simulink model "analysis1"  (Simulink 9.0)
settings: Solver=VariableStepAuto  StartTime=0.0  StopTime=0.1  RelTol=1e-3
libraries: dspstat3 x5
settings Model: Creator=CQC  LastModifiedBy=CQC
settings DataIOCC: SaveFormat=Dataset
settings OptimizationCC: LifeSpan=auto
settings DebuggingCC: UnderspecifiedInitializationDetection=Simplified  MergeDetectMultiDrivingBlocksExec=error  SFUnexpectedBacktrackingDiag=error  SFNoUnconditionalDefaultTransitionDiag=error  SFExecutionAtInitializationDiag=warning
settings HardwareCC: ProdBitPerPointer=64  ProdBitPerSizeT=64  ProdBitPerPtrDiffT=64  ProdLargestAtomicFloat=Float  ProdIntDivRoundTo=Zero  ProdEndianess=LittleEndian  ProdWordSize=64  ProdHWDeviceType=Intel->x86-64 (Windows64)
settings ModelReferenceCC: PropagateSignalLabelsOutOfModel=on
settings CodeAppCC: StateflowObjectComments=off
settings GRTTargetCC: TargetLangStandard=C99 (ISO)
settings ConfigComp: CovMetricSettings=dwe  CovHtmlReporting=off  CovSaveCumulativeToWorkspaceVar=off  CovSaveSingleToWorkspaceVar=off  CovExternalEMLEnable=on

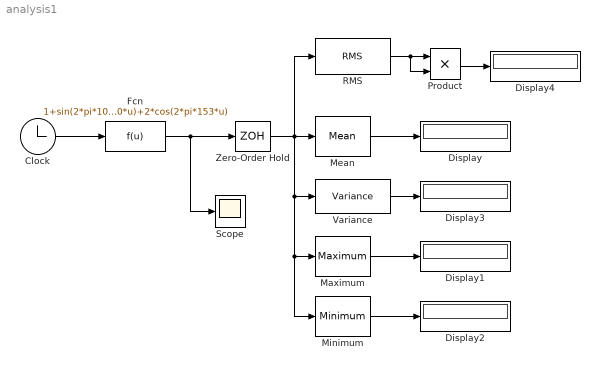
== system analysis1 ==
  Clock : Clock
      settings: Decimation=10000
  Display{,1..4} (5 alike) : Display
  Fcn : Fcn  Expr=1+sin(2*pi*100*u)+2*cos(2*pi*153*u)
  Maximum : dspstat3/Maximum  operation=maximum  fcn=Running  indexBase=One  operateOver=Each column  Dimension=1  InputProcessing=Columns as channels (frame based)  reset=None  roiEnable=off  roiType=Rectangles  roiPortion=Entire ROI  roiOutput=Individual statistics for each ROI  roiFlag=off  roundingMode=Floor  overflowMode=off  accumDataTypeStr=Inherit: Same as product output  accumLastDataTypeStr=Inherit: Same as product output
  Mean : dspstat3/Mean  run=on  reset_popup=None  InputProcessing=Columns as channels (frame based)  directionMode=Each column  dimension=1  roiEnable=off  roiType=Rectangles  roiPortion=Entire ROI  roiOutput=Individual statistics for each ROI  roiFlag=off  outputDataTypeStr=Inherit: Same as accumulator  outputLastDataTypeStr=Inherit: Same as accumulator  outputMin=[]  outputMax=[]  roundingMode=Floor  overflowMode=off
  Minimum : dspstat3/Minimum  operation=minimum  fcn=Running  indexBase=One  operateOver=Each column  Dimension=1  InputProcessing=Columns as channels (frame based)  reset=None  roiEnable=off  roiType=Rectangles  roiPortion=Entire ROI  roiOutput=Individual statistics for each ROI  roiFlag=off  roundingMode=Floor  overflowMode=off
      settings: SourceProductName=DSP System Toolbox  SourceProductBaseCode=DS
  Product : Product
  RMS : dspstat3/RMS  run=on  directionMode=Each column  dimension=1  InputProcessing=Columns as channels (frame based)  reset_popup=None
  Scope : Scope
  Variance : dspstat3/Variance  run=on  reset_popup=None  InputProcessing=Columns as channels (frame based)  directionMode=Each column  dimension=1  roiEnable=off  roiType=Rectangles  roiPortion=Entire ROI  roiOutput=Individual statistics for each ROI  roiFlag=off  roundingMode=Floor  overflowMode=off
      settings: SourceProductName=DSP System Toolbox
  Zero-Order Hold : ZeroOrderHold  SampleTime=-1
  wires:
  Clock/1 -> Fcn/1
  Fcn/1 -> Scope/1, Zero-Order Hold/1
  Zero-Order Hold/1 -> RMS/1, Variance/1, Maximum/1, Minimum/1, Mean/1
  Mean/1 -> Display/1
  Variance/1 -> Display3/1
  Minimum/1 -> Display2/1
  Maximum/1 -> Display1/1
  Product/1 -> Display4/1
  RMS/1 -> Product/2, Product/1
